simulink model "ss11"  (R2021b)
settings: Solver=ode23tb  StartTime=0.0  StopTime=25  FixedStep=1e-06  RelTol=1e-3  EnableMultiTasking=on
undefined symbols (not defined in the file): DiscIntNeverNeededParam, Par, sigbuilder_block, Ts
libraries: fl_lib x36, nesl_utility x30, ee_lib x12, simulink x9, simulink_extras x1, slpidlib x1
(part 2 of 2)

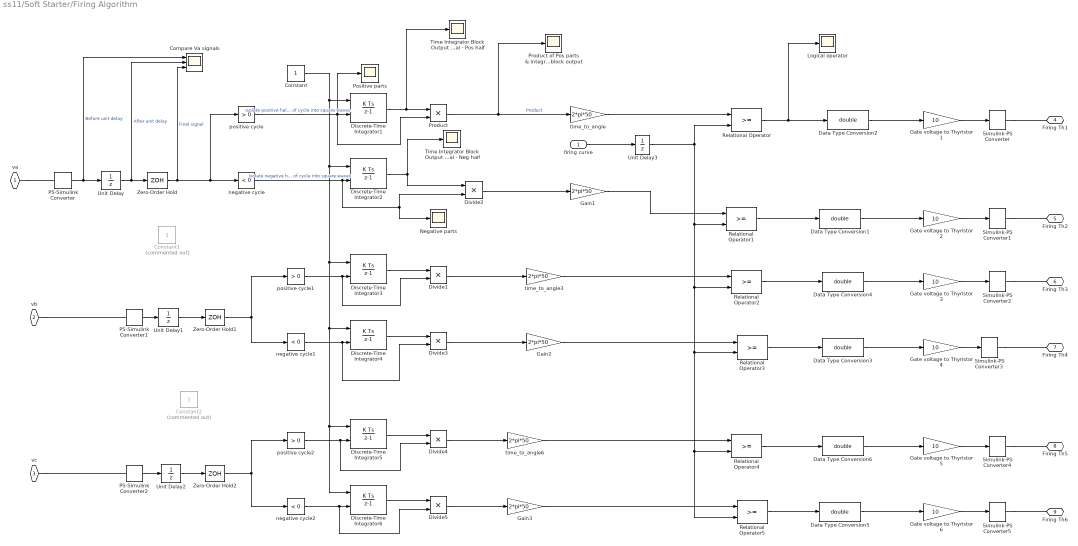
== system ss11/Soft Starter/Firing Algorithm ==
  firing curve : Inport
  Compare Va signals : Scope  NumInputPorts=3
  Constant : Constant  SampleTime=1.0e-04
  Constant1 : Constant  Commented=on  SampleTime=Ts
  Constant2 : Constant  Commented=on  SampleTime=Ts
  Data Type Conversion{1..6} (6 alike) : DataTypeConversion  OutDataTypeStr=double
  Discrete-Time Integrator{1..6} (6 alike) : DiscreteIntegrator  gainval=1  ExternalReset=rising  SampleTime=-1  ICPrevOutput=DiscIntNeverNeededParam  ICPrevScaledInput=DiscIntNeverNeededParam
  Divide{1..5} (5 alike) : Product  Inputs=**
  Gain1 : Gain  Gain=2*pi*50
  Gain2 : Gain  Gain=2*pi*50
  Gain3 : Gain  Gain=2*pi*50
  Gate voltage to Thyristor {1..6} (6 alike) : Gain  Gain=10
  Logical operator : Scope
  Negative parts : Scope
  PS-Simulink Converter : nesl_utility/PS-Simulink Converter  PhysicalDomain=network_engine_domain  SubClassName=ps_output  LeftPortType=input  RightPortType=output  PseudoPeriodic=off  Frequencies=[]  Unit=1  AffineConversion=off
      settings: SourceProductBaseCode=PW,SS
  PS-Simulink Converter1 : nesl_utility/PS-Simulink Converter  PhysicalDomain=network_engine_domain  SubClassName=ps_output  LeftPortType=input  RightPortType=output  PseudoPeriodic=off  Frequencies=[]  Unit=1  AffineConversion=off
      settings: SourceProductBaseCode=PW,SS
  PS-Simulink Converter2 : nesl_utility/PS-Simulink Converter  PhysicalDomain=network_engine_domain  SubClassName=ps_output  LeftPortType=input  RightPortType=output  PseudoPeriodic=off  Frequencies=[]  Unit=1  AffineConversion=off
      settings: SourceProductBaseCode=PW,SS
  Positive parts : Scope
  Product : Product
  Product of Pos parts & integrator block output : Scope
  Relational Operator{,1..5} (6 alike) : RelationalOperator  OutDataTypeStr=boolean  RndMeth=Nearest
  Simulink-PS Converter{,1..5} (6 alike) : nesl_utility/Simulink-PS Converter  PhysicalDomain=network_engine_domain  SubClassName=ps_input  LeftPortType=input  RightPortType=output  PseudoPeriodic=off  Frequencies=[]  NoiseDistribution=none  NoiseParameters=[]  Unit=V  AffineConversion=off  FilteringAndDerivatives=zero  SimscapeFilterOrder=1  InputFilterTimeConstant=0.001  UdotUserProvided=1
      settings: SourceProductBaseCode=PW,SS
  Time Integrator Block Output Signal - Neg half : Scope
  Time Integrator Block Output Signal - Pos half : Scope
  Unit Delay : UnitDelay  SampleTime=-1  HasFrameUpgradeWarning=on
  Unit Delay1 : UnitDelay  SampleTime=-1  HasFrameUpgradeWarning=on
  Unit Delay2 : UnitDelay  SampleTime=-1  HasFrameUpgradeWarning=on
  Unit Delay3 : UnitDelay  InitialCondition=5/6*pi  SampleTime=-1  HasFrameUpgradeWarning=on
  Zero-Order Hold : ZeroOrderHold  SampleTime=-1
  Zero-Order Hold1 : ZeroOrderHold  SampleTime=-1
  Zero-Order Hold2 : ZeroOrderHold  SampleTime=-1
  negative cycle : simulink/Logic and Bit Operations/Compare To Zero  relop=<  OutDataTypeStr=boolean
  negative cycle1 : simulink/Logic and Bit Operations/Compare To Zero  relop=<  OutDataTypeStr=boolean
  negative cycle2 : simulink/Logic and Bit Operations/Compare To Zero  relop=<  OutDataTypeStr=boolean
  positive cycle : simulink/Logic and Bit Operations/Compare To Zero  relop=>  OutDataTypeStr=boolean
  positive cycle1 : simulink/Logic and Bit Operations/Compare To Zero  relop=>  OutDataTypeStr=boolean
  positive cycle2 : simulink/Logic and Bit Operations/Compare To Zero  relop=>  OutDataTypeStr=boolean
  time_to_angle : Gain  Gain=2*pi*50
  time_to_angle3 : Gain  Gain=2*pi*50
  time_to_angle6 : Gain  Gain=2*pi*50
  va : PMIOPort  Side=Right
  vb : PMIOPort  Port=2  Side=Right
  vc : PMIOPort  Port=3  Side=Right
  Firing Th1 : PMIOPort  Port=4  Side=Left
  Firing Th2 : PMIOPort  Port=5  Side=Left
  Firing Th3 : PMIOPort  Port=6  Side=Left
  Firing Th4 : PMIOPort  Port=7  Side=Left
  Firing Th5 : PMIOPort  Port=8  Side=Left
  Firing Th6 : PMIOPort  Port=9  Side=Left
  wires:
  Discrete-Time Integrator1/1 -> Product/1, Time Integrator Block Output Signal - Pos half/1
  time_to_angle/1 -> Relational Operator/1
  Gain1/1 -> Relational Operator1/1
  negative cycle/1 -> Discrete-Time Integrator2/2, Negative parts/1, Divide2/2  "Isolate negative half of cycle into square waves"
  positive cycle/1 -> Product/2, Positive parts/1, Discrete-Time Integrator1/2  "Isolate positive half of cycle into square waves"
  Data Type Conversion1/1 -> Gate voltage to Thyristor 2/1
  Gate voltage to Thyristor 2/1 -> Simulink-PS Converter1/1
  Discrete-Time Integrator2/1 -> Time Integrator Block Output Signal - Neg half/1, Divide2/1
  Divide2/1 -> Gain1/1
  Product/1 -> Product of Pos parts & integrator block output/1, time_to_angle/1  "Product"
  Gate voltage to Thyristor 1/1 -> Simulink-PS Converter/1
  Data Type Conversion2/1 -> Gate voltage to Thyristor 1/1
  Relational Operator/1 -> Logical operator/1, Data Type Conversion2/1
  Relational Operator1/1 -> Data Type Conversion1/1
  Discrete-Time Integrator3/1 -> Divide1/1
  time_to_angle3/1 -> Relational Operator2/1
  Gain2/1 -> Relational Operator3/1
  negative cycle1/1 -> Discrete-Time Integrator4/2, Divide3/2
  positive cycle1/1 -> Divide1/2, Discrete-Time Integrator3/2
  Data Type Conversion3/1 -> Gate voltage to Thyristor 4/1
  Gate voltage to Thyristor 4/1 -> Simulink-PS Converter3/1
  Discrete-Time Integrator4/1 -> Divide3/1
  Divide3/1 -> Gain2/1
  Divide1/1 -> time_to_angle3/1
  Gate voltage to Thyristor 3/1 -> Simulink-PS Converter2/1
  Data Type Conversion4/1 -> Gate voltage to Thyristor 3/1
  Relational Operator2/1 -> Data Type Conversion4/1
  Relational Operator3/1 -> Data Type Conversion3/1
  Discrete-Time Integrator5/1 -> Divide4/1
  time_to_angle6/1 -> Relational Operator4/1
  Gain3/1 -> Relational Operator5/1
  negative cycle2/1 -> Divide5/2, Discrete-Time Integrator6/2
  positive cycle2/1 -> Divide4/2, Discrete-Time Integrator5/2
  Data Type Conversion5/1 -> Gate voltage to Thyristor 6/1
  Gate voltage to Thyristor 6/1 -> Simulink-PS Converter5/1
  Discrete-Time Integrator6/1 -> Divide5/1
  Divide5/1 -> Gain3/1
  Divide4/1 -> time_to_angle6/1
  Gate voltage to Thyristor 5/1 -> Simulink-PS Converter4/1
  Data Type Conversion6/1 -> Gate voltage to Thyristor 5/1
  Relational Operator4/1 -> Data Type Conversion6/1
  Relational Operator5/1 -> Data Type Conversion5/1
  PS-Simulink Converter1/1 -> Unit Delay1/1
  PS-Simulink Converter2/1 -> Unit Delay2/1
  firing curve/1 -> Unit Delay3/1
  PS-Simulink Converter/1 -> Unit Delay/1, Compare Va signals/1  "Before unit delay"
  Unit Delay/1 -> Compare Va signals/2, Zero-Order Hold/1  "After unit delay"
  Unit Delay1/1 -> Zero-Order Hold1/1
  Unit Delay2/1 -> Zero-Order Hold2/1
  Zero-Order Hold/1 -> negative cycle/1, positive cycle/1, Compare Va signals/3  "Final signal"
  Zero-Order Hold1/1 -> negative cycle1/1, positive cycle1/1
  Zero-Order Hold2/1 -> negative cycle2/1, positive cycle2/1
  Unit Delay3/1 -> Relational Operator5/2, Relational Operator4/2, Relational Operator3/2, Relational Operator2/2, Relational Operator1/2, Relational Operator/2
  Constant/1 -> Discrete-Time Integrator6/1, Discrete-Time Integrator5/1, Discrete-Time Integrator4/1, Discrete-Time Integrator3/1, Discrete-Time Integrator2/1, Discrete-Time Integrator1/1
  connections:
  Simulink-PS Converter1/RConn1 -- Firing Th2/RConn1
  Simulink-PS Converter/RConn1 -- Firing Th1/RConn1
  va/RConn1 -- PS-Simulink Converter/LConn1
  Simulink-PS Converter3/RConn1 -- Firing Th4/RConn1
  Simulink-PS Converter2/RConn1 -- Firing Th3/RConn1
  Simulink-PS Converter5/RConn1 -- Firing Th6/RConn1
  Simulink-PS Converter4/RConn1 -- Firing Th5/RConn1
  vb/RConn1 -- PS-Simulink Converter1/LConn1
  vc/RConn1 -- PS-Simulink Converter2/LConn1

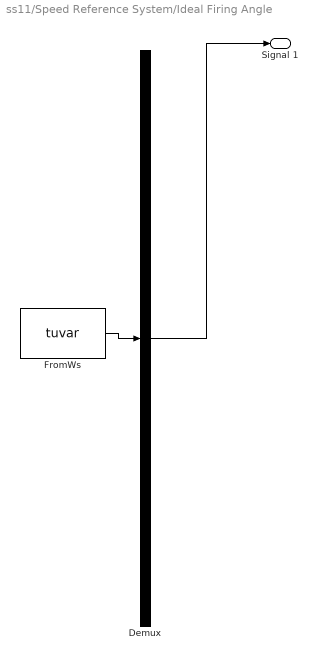
== system ss11/Speed Reference System/Ideal Firing Angle ==
  Demux : Demux  Tag=STV Demux  Outputs=1
      settings: DisplayOption=none
  FromWs : FromWorkspace  Tag=STV FromWs  VariableName=tuvar
      SigBuilderData=|
      | common.afterFinalStr = 'Extrapolate'
      | common.sampleTime = 0
      | dataSet.timeRange = [0 20]
      | dataSet.name = 'Group 1'
      | sbobj.Groups.Name = 'Group 1'
      | sbobj.Groups.Signals.Name = 'Signal 1'
      | sbobj.Groups.Signals.XData = [0 0.25 0.35 16 20]
      | sbobj.Groups.Signals.YData = [2.82743338823 2.86 2.86 0 0]
      | sbobj.Groups.TimeRange = [0 20]
  Signal 1 : Outport  Tag=STV Outport
  wires:
  Demux/1 -> Signal 1/1
  FromWs/1 -> Demux/1
